simulink model "top_uart"  (R2022b)
settings: Solver=FixedStepDiscrete  StartTime=0.0  StopTime=18e-5  RelTol=1e-3
undefined symbols (not defined in the file or in its folder): xc7a100tcsg324
libraries: vmcUtilities x1
settings Model: Creator=adiglesias  LastModifiedBy=adiglesias

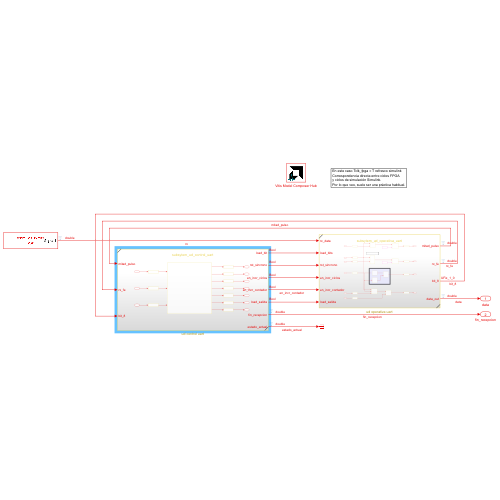
[thumbnail: Simulink's stored preview of the top-level diagram]
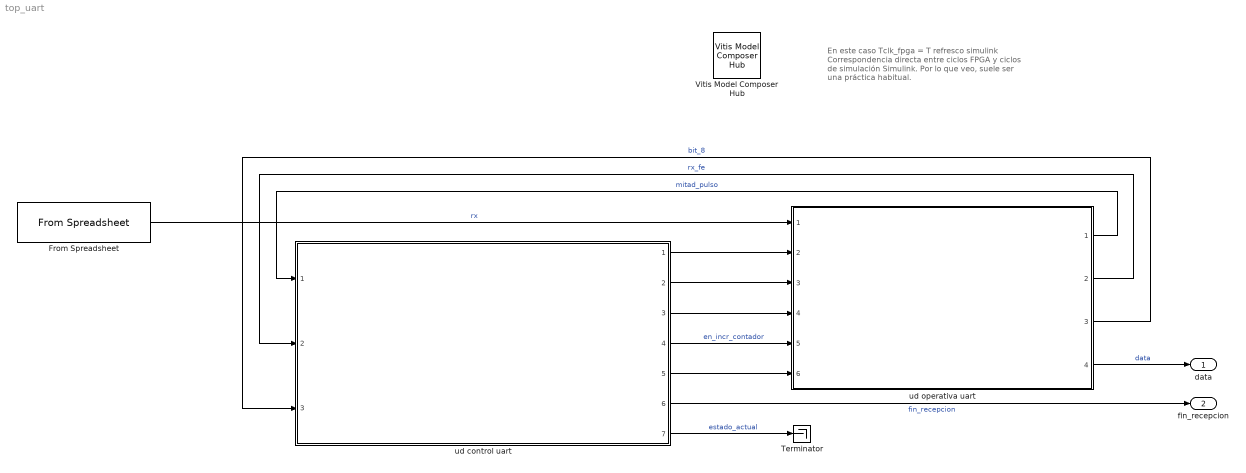
== system top_uart ==
  note: En este caso Tclk_fpga = T refresco simulink
      | Correspondencia directa entre ciclos FPGA
      | y ciclos de simulación Simulink.
      | Por lo que veo, suele ser una práctica habitual.
  From Spreadsheet : FromSpreadsheet  FileName=estimulos_rx.xlsx  SheetName=Hoja1  Range=A1:B46  SampleTime=10e-9
  Terminator : Terminator
  Vitis Model Composer Hub : vmcUtilities/Vitis Model Composer Hub  Tag=genX  CodeGeneration=off  SubsystemName=ud control uart  TargetDirectory=./code  ExportType=HDL  IpVendor=xilinx.com  IpLibrary=hls  IpVersion=1.0  IpHWLanguage=Verilog  AieCompilerOptions={}  AieSimulatorOptions={}  CreateTestbench=off  TestbenchStackSize=10  RunRtlSim=off  RunCSim=off  RunAieSim=off  AieSimTimeout=50000  RunAieSimProfiling=off  LaunchVitisAnalyzer=off  PlotOutput=off  RunX86Sim=off  X86SimTimeout=10  GenHwImage=off  GenLibadfXo=off  PlatformType=Not Specified  HwSystemType=Baremetal  HwValidationTarget=hw  ProjDevice=xc7a100tcsg324-1  ProjDevicePart=xc7a100tcsg324-1  AIEType=None  SamplePeriod=-1  ClockFrequency=200  DataPathParallelism=1  xilinxfamily=artix7  part=xc7a100t  speed=-1  package=csg324  directory=C:/Users/adiglesias/Desktop/code\ip\ud_control_uart\src  testbench=off  incr_netlist=off  synthesis_tool=Vivado  clock_wrapper=Clock Enables  dbl_ovrd=According to Block Masks  dcm_input_clock_period=10  sysclk_period=10  simulink_period=1/100e6  eval_field=0  IPInfoJsonString="{\"HDLSubsystem\":{\"SubsystemName\":\"ud_operativa_uart\",\"IPName\":\"ud_operativa_uart\",\"IPLibrary\":\"VMC\",\"IPVendor\":\"User Company\",\"IPVersion\":\"1.0\",\"TargetDirectory\":\"C:/Users/adiglesias/Desktop/code\",\"SubsystemDir\":\"C:/Users/adiglesias/Desktop/code\\\\ip\\\\ud_operativa_uart\"}}"  LogFileName=''  NThreads=4
  ud control uart : Subsystem  ReferencedSubsystem=subsytem_ud_control_uart
  ud operativa uart : Subsystem  ReferencedSubsystem=subsytem_ud_operativa_uart
  data : Outport
  fin_recepcion : Outport  Port=2
  wires:
  From Spreadsheet/1 -> ud operativa uart/1  "rx"
  ud control uart/1 -> ud operativa uart/2
  ud control uart/2 -> ud operativa uart/3
  ud control uart/3 -> ud operativa uart/4
  ud control uart/4 -> ud operativa uart/5  "en_incr_contador"
  ud operativa uart/1 -> ud control uart/1  "mitad_pulso"
  ud control uart/5 -> ud operativa uart/6
  ud control uart/6 -> fin_recepcion/1  "fin_recepcion"
  ud operativa uart/2 -> ud control uart/2  "rx_fe"
  ud operativa uart/3 -> ud control uart/3  "bit_8"
  ud operativa uart/4 -> data/1  "data"
  ud control uart/7 -> Terminator/1  "estado_actual"
